simulink model "nonlinear"  (R2024a)
settings: Solver=ode45  StartTime=0.0  StopTime=50  RelTol=1e-3
values from neighbouring files (symbols this model uses):
  K = in(1:2)    [controller.m]    (also in init.m = [30 10])
  x10 = 1    [init.m]
  x20 = 1    [init.m]
settings Model: Creator=Melkamu A  LastModifiedBy=Melkamu A
settings SolverCC: MaxConsecutiveMinStep=3  AlgebraicLoopSolver=LineSearch
settings DebuggingCC: UnconnectedInputMsg=warning  UnconnectedOutputMsg=warning  UnconnectedLineMsg=warning
settings ModelReferenceCC: EnableRefExpFcnMdlSchedulingChecks=on
settings RTWCC: GPUComputeCapability=3.5  DLArmComputeVersion=19.05

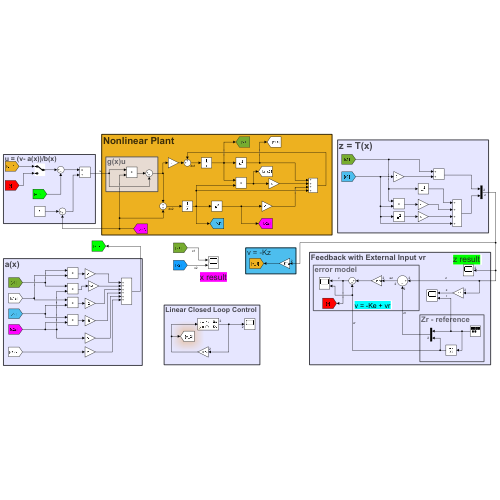
[thumbnail: Simulink's stored preview of the top-level diagram]
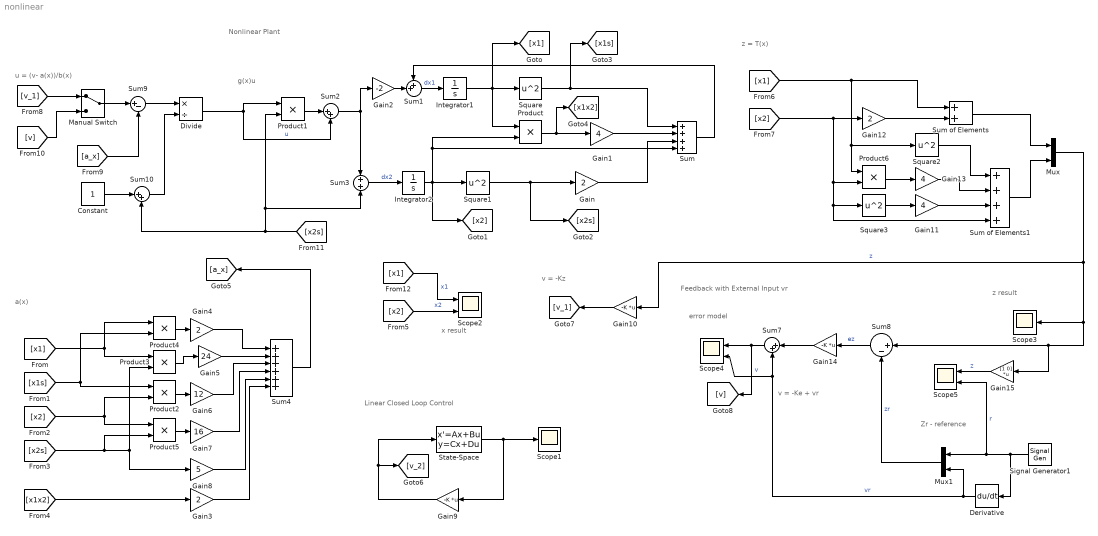
== system nonlinear ==
  note: v = -Kz
  note: g(x)u
  note: Feedback with External Input vr
  note: u = (v- a(x))/b(x)
  note: Linear Closed Loop Control
  note: a(x)
  note: z = T(x)
  note: Nonlinear Plant
  note: Zr - reference
  note: error model
  note: z result
  note: x result
  note: v = -Ke + vr
  Constant : Constant
  Derivative : Derivative
  Divide : Product  Inputs=*/
  Gain{,3..4,12} (4 alike) : Gain  Gain=2
  Gain1 : Gain  Gain=4
  Gain10 : Gain  Gain=-K  Multiplication=Matrix(K*u)
  Gain11 : Gain  Gain=4
  Gain13 : Gain  Gain=4
  Gain14 : Gain  Gain=-K  Multiplication=Matrix(K*u)
  Gain15 : Gain  Gain=[1 0]  Multiplication=Matrix(K*u)
  Gain2 : Gain  Gain=-2
  Gain5 : Gain  Gain=24
  Gain6 : Gain  Gain=12
  Gain7 : Gain  Gain=16
  Gain8 : Gain  Gain=5
  Gain9 : Gain  Gain=-K  Multiplication=Matrix(K*u)
  Integrator1 : Integrator  InitialCondition=x10  UpperSaturationLimit=100  LowerSaturationLimit=-10
  Integrator2 : Integrator  InitialCondition=x20  UpperSaturationLimit=10  LowerSaturationLimit=-100
  Manual Switch : ManualSwitch
  Mux : Mux  Inputs=2
  Mux1 : Mux  Inputs=2
  Product{,1..6} (7 alike) : Product
  Scope1 : Scope
  Scope2 : Scope  NumInputPorts=2
  Scope3 : Scope
  Scope4 : Scope  NumInputPorts=2
  Scope5 : Scope  NumInputPorts=2
  Signal Generator1 : SignalGenerator  Amplitude=2  Frequency=0.2  Units=rad/sec
  Square{,1..3} (4 alike) : Math  Operator=square
  State-Space : StateSpace  A=[0 1; 0 0]  B=[0; 1]  C=[1 0; 0 1]  D=[0; 0]  InitialCondition=[x10; x20]
  Sum : Sum  Inputs=++++
  Sum of Elements : Sum
  Sum of Elements1 : Sum  Inputs=++++
  Sum1 : Sum  Inputs=++|
  Sum10 : Sum  Inputs=|++
  Sum2 : Sum  Inputs=|++
  Sum3 : Sum
  Sum4 : Sum  Inputs=++++++
  Sum7 : Sum  Inputs=|++
  Sum8 : Sum  Inputs=|+-
  Sum9 : Sum  Inputs=|+-
  wires:
  Integrator1/1 -> [x1], Square/1, Product/1
  Sum1/1 -> Integrator1/1  "dx1"
  Gain/1 -> Sum/3
  Square/1 -> [x1s], Sum/1
  Sum3/1 -> Integrator2/1  "dx2"
  Gain1/1 -> Sum/2
  Product/1 -> [x1x2], Gain1/1
  Integrator2/1 -> [x2], Square1/1, Sum/4, Product/2
  Gain2/1 -> Sum1/2
  Product6/1 -> Gain13/1
  Gain12/1 -> Sum of Elements/2
  [x1] -> Sum of Elements/1, Square2/1, Product6/1
  Gain13/1 -> Sum of Elements1/2
  Square2/1 -> Sum of Elements1/1
  Gain11/1 -> Sum of Elements1/3
  Sum of Elements1/1 -> Mux/2
  Sum of Elements/1 -> Mux/1
  [x2] -> Gain12/1, Product6/2, Sum of Elements1/4, Square3/1
  Square3/1 -> Gain11/1
  Gain5/1 -> Sum4/2
  Gain7/1 -> Sum4/4
  Gain8/1 -> Sum4/5
  Product3/1 -> Gain5/1
  [x2] -> Product5/1, Product2/2
  Gain3/1 -> Sum4/6
  [x1s] -> Product2/1, Product4/2
  [x1x2] -> Gain3/1
  Gain6/1 -> Sum4/3
  Product2/1 -> Gain6/1
  Product4/1 -> Gain4/1
  [x2s] -> Product3/2, Gain8/1, Product5/2
  [x1] -> Product4/1, Product3/1
  Product5/1 -> Gain7/1
  Gain4/1 -> Sum4/1
  Sum4/1 -> [a_x]
  Sum/1 -> Sum1/1
  Mux/1 -> Gain10/1, Gain15/1, Sum8/1, Scope3/1  "z"
  State-Space/1 -> Scope1/1, Gain9/1
  [v_1] -> Manual Switch/1
  Constant/1 -> Sum10/1
  Divide/1 -> Sum2/2, Product1/1  "u"
  [a_x] -> Sum9/2
  Sum10/1 -> Divide/2
  Sum9/1 -> Divide/1
  Gain14/1 -> Sum7/1
  Sum7/1 -> Scope4/1, [v]  "v"
  Sum8/1 -> Gain14/1  "ez"
  Derivative/1 -> Mux1/2, Sum7/2, Scope4/2  "vr"
  Mux1/1 -> Sum8/2  "zr"
  Signal Generator1/1 -> Scope5/2, Mux1/1, Derivative/1  "r"
  Manual Switch/1 -> Sum9/1
  [v] -> Manual Switch/2
  Sum2/1 -> Gain2/1, Sum3/1
  Square1/1 -> [x2s], Gain/1
  Product1/1 -> Sum2/1
  [x2s] -> Product1/2, Sum3/2, Sum10/2
  [x2] -> Scope2/2  "x2"
  [x1] -> Scope2/1  "x1"
  Gain10/1 -> [v_1]
  Gain9/1 -> [v_2], State-Space/1
  Gain15/1 -> Scope5/1  "z"
